simulink model "cichbcic_core"  (Simulink 7.9)
settings: Solver=ode45  StartTime=0.0  StopTime=10.0  RelTol=1e-3
libraries: xbsIndex_r4 x375
(part 2 of 5)

== system cichbcic_core/cic_stage_dec4/adder_tree1 ==
  sync : Inport
  din_1 : Inport  Port=2
  din_2 : Inport  Port=3
  adder_0 : xbsIndex_r4/AddSub  mode=Addition  use_carryin=off  use_carryout=off  en=off  latency=4  precision=Full  arith_type=Unsigned  n_bits=18  bin_pt=17  quantization="Round  (unbiased: +/- Inf)"  overflow=Saturate  dbl_ovrd=off  use_behavioral_HDL=on  hw_selection=Fabric  pipelined=off  block_type=addsub
  sync_delay : xbsIndex_r4/Delay  rst=off  infoeditControl=Selection of Reset will increase slice count due to use of real FFs and instead of SRLs  en=off  latency=4  dbl_ovrd=off  reg_retiming=off  block_type=delay
  sync_out : Outport
  dout : Outport  Port=2
  wires:
  sync/1 -> sync_delay/1
  sync_delay/1 -> sync_out/1
  din_2/1 -> adder_0/1
  din_1/1 -> adder_0/2
  adder_0/1 -> dout/1

== system cichbcic_core/cic_stage_dec4/adder_tree2 ==
  sync : Inport
  din_1 : Inport  Port=2
  din_2 : Inport  Port=3
  adder_0 : xbsIndex_r4/AddSub  mode=Addition  use_carryin=off  use_carryout=off  en=off  latency=4  precision=Full  arith_type=Unsigned  n_bits=18  bin_pt=17  quantization="Round  (unbiased: +/- Inf)"  overflow=Saturate  dbl_ovrd=off  use_behavioral_HDL=on  hw_selection=Fabric  pipelined=off  block_type=addsub
  sync_delay : xbsIndex_r4/Delay  rst=off  infoeditControl=Selection of Reset will increase slice count due to use of real FFs and instead of SRLs  en=off  latency=4  dbl_ovrd=off  reg_retiming=off  block_type=delay
  sync_out : Outport
  dout : Outport  Port=2
  wires:
  sync/1 -> sync_delay/1
  sync_delay/1 -> sync_out/1
  din_2/1 -> adder_0/1
  din_1/1 -> adder_0/2
  adder_0/1 -> dout/1

== system cichbcic_core/cic_stage_dec4/adder_tree3 ==
  sync : Inport
  din_1 : Inport  Port=2
  din_2 : Inport  Port=3
  adder_0 : xbsIndex_r4/AddSub  mode=Addition  use_carryin=off  use_carryout=off  en=off  latency=4  precision=Full  arith_type=Unsigned  n_bits=18  bin_pt=17  quantization="Round  (unbiased: +/- Inf)"  overflow=Saturate  dbl_ovrd=off  use_behavioral_HDL=on  hw_selection=Fabric  pipelined=off  block_type=addsub
  sync_delay : xbsIndex_r4/Delay  rst=off  infoeditControl=Selection of Reset will increase slice count due to use of real FFs and instead of SRLs  en=off  latency=4  dbl_ovrd=off  reg_retiming=off  block_type=delay
  sync_out : Outport
  dout : Outport  Port=2
  wires:
  sync/1 -> sync_delay/1
  sync_delay/1 -> sync_out/1
  din_2/1 -> adder_0/1
  din_1/1 -> adder_0/2
  adder_0/1 -> dout/1

== system cichbcic_core/Halfband1/adder_tree/addr1 ==
  data_a : Inport
  data_b : Inport  Port=2
  en_in : Inport  Port=3
  AddSub : xbsIndex_r4/AddSub  mode=Addition  use_carryin=off  use_carryout=off  en=on  latency=2  precision=Full  arith_type=Unsigned  n_bits=16  bin_pt=14  quantization=Truncate  overflow=Wrap  dbl_ovrd=off  use_behavioral_HDL=off  hw_selection=Fabric  pipelined=off  block_type=addsub
  sum_ab : Outport
  en_out : Outport  Port=2
  wires:
  data_b/1 -> AddSub/1
  data_a/1 -> AddSub/2
  en_in/1 -> AddSub/3, en_out/1
  AddSub/1 -> sum_ab/1

== system cichbcic_core/Halfband1/adder_tree/addr11 ==
  data_a : Inport
  data_b : Inport  Port=2
  en_in : Inport  Port=3
  AddSub : xbsIndex_r4/AddSub  mode=Addition  use_carryin=off  use_carryout=off  en=on  latency=2  precision=Full  arith_type=Unsigned  n_bits=16  bin_pt=14  quantization=Truncate  overflow=Wrap  dbl_ovrd=off  use_behavioral_HDL=off  hw_selection=Fabric  pipelined=off  block_type=addsub
  sum_ab : Outport
  en_out : Outport  Port=2
  wires:
  data_b/1 -> AddSub/1
  data_a/1 -> AddSub/2
  en_in/1 -> AddSub/3, en_out/1
  AddSub/1 -> sum_ab/1

== system cichbcic_core/Halfband1/adder_tree/addr2 ==
  data_a : Inport
  data_b : Inport  Port=2
  en_in : Inport  Port=3
  AddSub : xbsIndex_r4/AddSub  mode=Addition  use_carryin=off  use_carryout=off  en=on  latency=2  precision=Full  arith_type=Unsigned  n_bits=16  bin_pt=14  quantization=Truncate  overflow=Wrap  dbl_ovrd=off  use_behavioral_HDL=off  hw_selection=Fabric  pipelined=off  block_type=addsub
  sum_ab : Outport
  en_out : Outport  Port=2
  wires:
  data_b/1 -> AddSub/1
  data_a/1 -> AddSub/2
  en_in/1 -> AddSub/3, en_out/1
  AddSub/1 -> sum_ab/1

== system cichbcic_core/Halfband1/adder_tree/addr3 ==
  data_a : Inport
  data_b : Inport  Port=2
  en_in : Inport  Port=3
  AddSub : xbsIndex_r4/AddSub  mode=Addition  use_carryin=off  use_carryout=off  en=on  latency=2  precision=Full  arith_type=Unsigned  n_bits=16  bin_pt=14  quantization=Truncate  overflow=Wrap  dbl_ovrd=off  use_behavioral_HDL=off  hw_selection=Fabric  pipelined=off  block_type=addsub
  sum_ab : Outport
  en_out : Outport  Port=2
  wires:
  data_b/1 -> AddSub/1
  data_a/1 -> AddSub/2
  en_in/1 -> AddSub/3, en_out/1
  AddSub/1 -> sum_ab/1

== system cichbcic_core/Halfband1/adder_tree/addr4 ==
  data_a : Inport
  data_b : Inport  Port=2
  en_in : Inport  Port=3
  AddSub : xbsIndex_r4/AddSub  mode=Addition  use_carryin=off  use_carryout=off  en=on  latency=2  precision=Full  arith_type=Unsigned  n_bits=16  bin_pt=14  quantization=Truncate  overflow=Wrap  dbl_ovrd=off  use_behavioral_HDL=off  hw_selection=Fabric  pipelined=off  block_type=addsub
  sum_ab : Outport
  en_out : Outport  Port=2
  wires:
  data_b/1 -> AddSub/1
  data_a/1 -> AddSub/2
  en_in/1 -> AddSub/3, en_out/1
  AddSub/1 -> sum_ab/1

== system cichbcic_core/Halfband1/adder_tree/addr6 ==
  data_a : Inport
  data_b : Inport  Port=2
  en_in : Inport  Port=3
  AddSub : xbsIndex_r4/AddSub  mode=Addition  use_carryin=off  use_carryout=off  en=on  latency=2  precision=Full  arith_type=Unsigned  n_bits=16  bin_pt=14  quantization=Truncate  overflow=Wrap  dbl_ovrd=off  use_behavioral_HDL=off  hw_selection=Fabric  pipelined=off  block_type=addsub
  sum_ab : Outport
  en_out : Outport  Port=2
  wires:
  data_b/1 -> AddSub/1
  data_a/1 -> AddSub/2
  en_in/1 -> AddSub/3, en_out/1
  AddSub/1 -> sum_ab/1

== system cichbcic_core/Halfband1/adder_tree/addr7 ==
  data_a : Inport
  data_b : Inport  Port=2
  en_in : Inport  Port=3
  AddSub : xbsIndex_r4/AddSub  mode=Addition  use_carryin=off  use_carryout=off  en=on  latency=2  precision=Full  arith_type=Unsigned  n_bits=16  bin_pt=14  quantization=Truncate  overflow=Wrap  dbl_ovrd=off  use_behavioral_HDL=off  hw_selection=Fabric  pipelined=off  block_type=addsub
  sum_ab : Outport
  en_out : Outport  Port=2
  wires:
  data_b/1 -> AddSub/1
  data_a/1 -> AddSub/2
  en_in/1 -> AddSub/3, en_out/1
  AddSub/1 -> sum_ab/1

== system cichbcic_core/Halfband1/adder_tree/addr9 ==
  data_a : Inport
  data_b : Inport  Port=2
  en_in : Inport  Port=3
  AddSub : xbsIndex_r4/AddSub  mode=Addition  use_carryin=off  use_carryout=off  en=on  latency=2  precision=Full  arith_type=Unsigned  n_bits=16  bin_pt=14  quantization=Truncate  overflow=Wrap  dbl_ovrd=off  use_behavioral_HDL=off  hw_selection=Fabric  pipelined=off  block_type=addsub
  sum_ab : Outport
  en_out : Outport  Port=2
  wires:
  data_b/1 -> AddSub/1
  data_a/1 -> AddSub/2
  en_in/1 -> AddSub/3, en_out/1
  AddSub/1 -> sum_ab/1

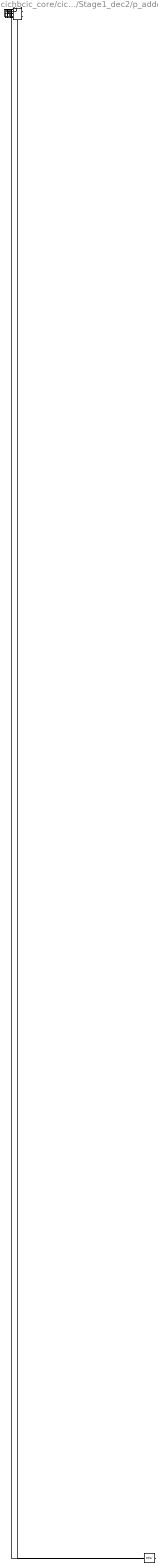
== system cichbcic_core/cic_pow2_1/Stage1_dec2/p_adder1 ==
  sync_in : Inport
  in1 : Inport  Port=2
  in2 : Inport  Port=3
  in3 : Inport  Port=4
  in4 : Inport  Port=5
  in5 : Inport  Port=6
  in6 : Inport  Port=7
  in7 : Inport  Port=8
  in8 : Inport  Port=9
  in9 : Inport  Port=10
  in10 : Inport  Port=11
  in11 : Inport  Port=12
  in12 : Inport  Port=13
  in13 : Inport  Port=14
  in14 : Inport  Port=15
  in15 : Inport  Port=16
  in16 : Inport  Port=17
  adder_tree1 : Subsystem
  adder_tree10 : Subsystem
  adder_tree11 : Subsystem
  adder_tree12 : Subsystem
  adder_tree13 : Subsystem
  adder_tree14 : Subsystem
  adder_tree15 : Subsystem
  adder_tree16 : Subsystem
  adder_tree2 : Subsystem
  adder_tree3 : Subsystem
  adder_tree4 : Subsystem
  adder_tree5 : Subsystem
  adder_tree6 : Subsystem
  adder_tree7 : Subsystem
  adder_tree8 : Subsystem
  adder_tree9 : Subsystem
  delay16 : xbsIndex_r4/Delay  rst=off  infoeditControl=Selection of Reset will increase slice count due to use of real FFs and instead of SRLs  en=off  latency=1  dbl_ovrd=off  reg_retiming=off  block_type=delay
  sync_out : Outport
  out1 : Outport  Port=2
  out2 : Outport  Port=3
  out3 : Outport  Port=4
  out4 : Outport  Port=5
  out5 : Outport  Port=6
  out6 : Outport  Port=7
  out7 : Outport  Port=8
  out8 : Outport  Port=9
  out9 : Outport  Port=10
  out10 : Outport  Port=11
  out11 : Outport  Port=12
  out12 : Outport  Port=13
  out13 : Outport  Port=14
  out14 : Outport  Port=15
  out15 : Outport  Port=16
  out16 : Outport  Port=17
  wires:
  in16/1 -> delay16/1, adder_tree16/2(din_1)
  sync_in/1 -> adder_tree1/1(sync)
  in1/1 -> adder_tree1/2(din_1), adder_tree2/3(din_2)
  delay16/1 -> adder_tree1/3(din_2)  "d16"
  adder_tree1/2(dout) -> out1/1
  adder_tree1/1(sync_out) -> adder_tree2/1(sync)  "adder_tree_sync_in1"
  in2/1 -> adder_tree2/2(din_1), adder_tree3/3(din_2)
  adder_tree2/2(dout) -> out2/1
  adder_tree2/1(sync_out) -> adder_tree3/1(sync)  "adder_tree_sync_in2"
  in3/1 -> adder_tree3/2(din_1), adder_tree4/3(din_2)
  adder_tree3/2(dout) -> out3/1
  adder_tree3/1(sync_out) -> adder_tree4/1(sync)  "adder_tree_sync_in3"
  in4/1 -> adder_tree4/2(din_1), adder_tree5/3(din_2)
  adder_tree4/2(dout) -> out4/1
  adder_tree4/1(sync_out) -> adder_tree5/1(sync)  "adder_tree_sync_in4"
  in5/1 -> adder_tree5/2(din_1), adder_tree6/3(din_2)
  adder_tree5/2(dout) -> out5/1
  adder_tree5/1(sync_out) -> adder_tree6/1(sync)  "adder_tree_sync_in5"
  in6/1 -> adder_tree6/2(din_1), adder_tree7/3(din_2)
  adder_tree6/2(dout) -> out6/1
  adder_tree6/1(sync_out) -> adder_tree7/1(sync)  "adder_tree_sync_in6"
  in7/1 -> adder_tree7/2(din_1), adder_tree8/3(din_2)
  adder_tree7/2(dout) -> out7/1
  adder_tree7/1(sync_out) -> adder_tree8/1(sync)  "adder_tree_sync_in7"
  in8/1 -> adder_tree8/2(din_1), adder_tree9/3(din_2)
  adder_tree8/2(dout) -> out8/1
  adder_tree8/1(sync_out) -> adder_tree9/1(sync)  "adder_tree_sync_in8"
  in9/1 -> adder_tree9/2(din_1), adder_tree10/3(din_2)
  adder_tree9/2(dout) -> out9/1
  adder_tree9/1(sync_out) -> adder_tree10/1(sync)  "adder_tree_sync_in9"
  in10/1 -> adder_tree10/2(din_1), adder_tree11/3(din_2)
  adder_tree10/2(dout) -> out10/1
  adder_tree10/1(sync_out) -> adder_tree11/1(sync)  "adder_tree_sync_in10"
  in11/1 -> adder_tree11/2(din_1), adder_tree12/3(din_2)
  adder_tree11/2(dout) -> out11/1
  adder_tree11/1(sync_out) -> adder_tree12/1(sync)  "adder_tree_sync_in11"
  in12/1 -> adder_tree12/2(din_1), adder_tree13/3(din_2)
  adder_tree12/2(dout) -> out12/1
  adder_tree12/1(sync_out) -> adder_tree13/1(sync)  "adder_tree_sync_in12"
  in13/1 -> adder_tree13/2(din_1), adder_tree14/3(din_2)
  adder_tree13/2(dout) -> out13/1
  adder_tree13/1(sync_out) -> adder_tree14/1(sync)  "adder_tree_sync_in13"
  in14/1 -> adder_tree14/2(din_1), adder_tree15/3(din_2)
  adder_tree14/2(dout) -> out14/1
  adder_tree14/1(sync_out) -> adder_tree15/1(sync)  "adder_tree_sync_in14"
  in15/1 -> adder_tree15/2(din_1), adder_tree16/3(din_2)
  adder_tree15/2(dout) -> out15/1
  adder_tree15/1(sync_out) -> adder_tree16/1(sync)  "adder_tree_sync_in15"
  adder_tree16/2(dout) -> out16/1
  adder_tree16/1(sync_out) -> sync_out/1  "adder_tree_sync_in16"

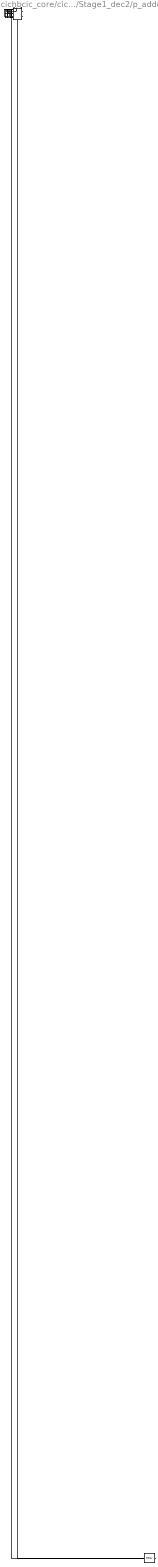
== system cichbcic_core/cic_pow2_1/Stage1_dec2/p_adder2 ==
  sync_in : Inport
  in1 : Inport  Port=2
  in2 : Inport  Port=3
  in3 : Inport  Port=4
  in4 : Inport  Port=5
  in5 : Inport  Port=6
  in6 : Inport  Port=7
  in7 : Inport  Port=8
  in8 : Inport  Port=9
  in9 : Inport  Port=10
  in10 : Inport  Port=11
  in11 : Inport  Port=12
  in12 : Inport  Port=13
  in13 : Inport  Port=14
  in14 : Inport  Port=15
  in15 : Inport  Port=16
  in16 : Inport  Port=17
  adder_tree1 : Subsystem
  adder_tree10 : Subsystem
  adder_tree11 : Subsystem
  adder_tree12 : Subsystem
  adder_tree13 : Subsystem
  adder_tree14 : Subsystem
  adder_tree15 : Subsystem
  adder_tree16 : Subsystem
  adder_tree2 : Subsystem
  adder_tree3 : Subsystem
  adder_tree4 : Subsystem
  adder_tree5 : Subsystem
  adder_tree6 : Subsystem
  adder_tree7 : Subsystem
  adder_tree8 : Subsystem
  adder_tree9 : Subsystem
  delay16 : xbsIndex_r4/Delay  rst=off  infoeditControl=Selection of Reset will increase slice count due to use of real FFs and instead of SRLs  en=off  latency=1  dbl_ovrd=off  reg_retiming=off  block_type=delay
  sync_out : Outport
  out1 : Outport  Port=2
  out2 : Outport  Port=3
  out3 : Outport  Port=4
  out4 : Outport  Port=5
  out5 : Outport  Port=6
  out6 : Outport  Port=7
  out7 : Outport  Port=8
  out8 : Outport  Port=9
  out9 : Outport  Port=10
  out10 : Outport  Port=11
  out11 : Outport  Port=12
  out12 : Outport  Port=13
  out13 : Outport  Port=14
  out14 : Outport  Port=15
  out15 : Outport  Port=16
  out16 : Outport  Port=17
  wires:
  in16/1 -> delay16/1, adder_tree16/2(din_1)
  sync_in/1 -> adder_tree1/1(sync)
  in1/1 -> adder_tree1/2(din_1), adder_tree2/3(din_2)
  delay16/1 -> adder_tree1/3(din_2)  "d16"
  adder_tree1/2(dout) -> out1/1
  adder_tree1/1(sync_out) -> adder_tree2/1(sync)  "adder_tree_sync_in1"
  in2/1 -> adder_tree2/2(din_1), adder_tree3/3(din_2)
  adder_tree2/2(dout) -> out2/1
  adder_tree2/1(sync_out) -> adder_tree3/1(sync)  "adder_tree_sync_in2"
  in3/1 -> adder_tree3/2(din_1), adder_tree4/3(din_2)
  adder_tree3/2(dout) -> out3/1
  adder_tree3/1(sync_out) -> adder_tree4/1(sync)  "adder_tree_sync_in3"
  in4/1 -> adder_tree4/2(din_1), adder_tree5/3(din_2)
  adder_tree4/2(dout) -> out4/1
  adder_tree4/1(sync_out) -> adder_tree5/1(sync)  "adder_tree_sync_in4"
  in5/1 -> adder_tree5/2(din_1), adder_tree6/3(din_2)
  adder_tree5/2(dout) -> out5/1
  adder_tree5/1(sync_out) -> adder_tree6/1(sync)  "adder_tree_sync_in5"
  in6/1 -> adder_tree6/2(din_1), adder_tree7/3(din_2)
  adder_tree6/2(dout) -> out6/1
  adder_tree6/1(sync_out) -> adder_tree7/1(sync)  "adder_tree_sync_in6"
  in7/1 -> adder_tree7/2(din_1), adder_tree8/3(din_2)
  adder_tree7/2(dout) -> out7/1
  adder_tree7/1(sync_out) -> adder_tree8/1(sync)  "adder_tree_sync_in7"
  in8/1 -> adder_tree8/2(din_1), adder_tree9/3(din_2)
  adder_tree8/2(dout) -> out8/1
  adder_tree8/1(sync_out) -> adder_tree9/1(sync)  "adder_tree_sync_in8"
  in9/1 -> adder_tree9/2(din_1), adder_tree10/3(din_2)
  adder_tree9/2(dout) -> out9/1
  adder_tree9/1(sync_out) -> adder_tree10/1(sync)  "adder_tree_sync_in9"
  in10/1 -> adder_tree10/2(din_1), adder_tree11/3(din_2)
  adder_tree10/2(dout) -> out10/1
  adder_tree10/1(sync_out) -> adder_tree11/1(sync)  "adder_tree_sync_in10"
  in11/1 -> adder_tree11/2(din_1), adder_tree12/3(din_2)
  adder_tree11/2(dout) -> out11/1
  adder_tree11/1(sync_out) -> adder_tree12/1(sync)  "adder_tree_sync_in11"
  in12/1 -> adder_tree12/2(din_1), adder_tree13/3(din_2)
  adder_tree12/2(dout) -> out12/1
  adder_tree12/1(sync_out) -> adder_tree13/1(sync)  "adder_tree_sync_in12"
  in13/1 -> adder_tree13/2(din_1), adder_tree14/3(din_2)
  adder_tree13/2(dout) -> out13/1
  adder_tree13/1(sync_out) -> adder_tree14/1(sync)  "adder_tree_sync_in13"
  in14/1 -> adder_tree14/2(din_1), adder_tree15/3(din_2)
  adder_tree14/2(dout) -> out14/1
  adder_tree14/1(sync_out) -> adder_tree15/1(sync)  "adder_tree_sync_in14"
  in15/1 -> adder_tree15/2(din_1), adder_tree16/3(din_2)
  adder_tree15/2(dout) -> out15/1
  adder_tree15/1(sync_out) -> adder_tree16/1(sync)  "adder_tree_sync_in15"
  adder_tree16/2(dout) -> out16/1
  adder_tree16/1(sync_out) -> sync_out/1  "adder_tree_sync_in16"

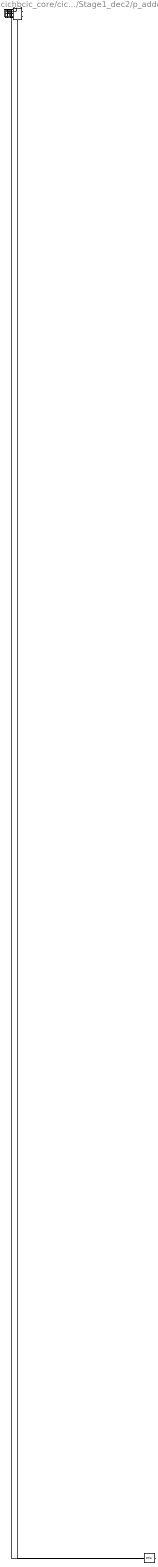
== system cichbcic_core/cic_pow2_1/Stage1_dec2/p_adder3 ==
  sync_in : Inport
  in1 : Inport  Port=2
  in2 : Inport  Port=3
  in3 : Inport  Port=4
  in4 : Inport  Port=5
  in5 : Inport  Port=6
  in6 : Inport  Port=7
  in7 : Inport  Port=8
  in8 : Inport  Port=9
  in9 : Inport  Port=10
  in10 : Inport  Port=11
  in11 : Inport  Port=12
  in12 : Inport  Port=13
  in13 : Inport  Port=14
  in14 : Inport  Port=15
  in15 : Inport  Port=16
  in16 : Inport  Port=17
  adder_tree1 : Subsystem
  adder_tree10 : Subsystem
  adder_tree11 : Subsystem
  adder_tree12 : Subsystem
  adder_tree13 : Subsystem
  adder_tree14 : Subsystem
  adder_tree15 : Subsystem
  adder_tree16 : Subsystem
  adder_tree2 : Subsystem
  adder_tree3 : Subsystem
  adder_tree4 : Subsystem
  adder_tree5 : Subsystem
  adder_tree6 : Subsystem
  adder_tree7 : Subsystem
  adder_tree8 : Subsystem
  adder_tree9 : Subsystem
  delay16 : xbsIndex_r4/Delay  rst=off  infoeditControl=Selection of Reset will increase slice count due to use of real FFs and instead of SRLs  en=off  latency=1  dbl_ovrd=off  reg_retiming=off  block_type=delay
  sync_out : Outport
  out1 : Outport  Port=2
  out2 : Outport  Port=3
  out3 : Outport  Port=4
  out4 : Outport  Port=5
  out5 : Outport  Port=6
  out6 : Outport  Port=7
  out7 : Outport  Port=8
  out8 : Outport  Port=9
  out9 : Outport  Port=10
  out10 : Outport  Port=11
  out11 : Outport  Port=12
  out12 : Outport  Port=13
  out13 : Outport  Port=14
  out14 : Outport  Port=15
  out15 : Outport  Port=16
  out16 : Outport  Port=17
  wires:
  in16/1 -> delay16/1, adder_tree16/2(din_1)
  sync_in/1 -> adder_tree1/1(sync)
  in1/1 -> adder_tree1/2(din_1), adder_tree2/3(din_2)
  delay16/1 -> adder_tree1/3(din_2)  "d16"
  adder_tree1/2(dout) -> out1/1
  adder_tree1/1(sync_out) -> adder_tree2/1(sync)  "adder_tree_sync_in1"
  in2/1 -> adder_tree2/2(din_1), adder_tree3/3(din_2)
  adder_tree2/2(dout) -> out2/1
  adder_tree2/1(sync_out) -> adder_tree3/1(sync)  "adder_tree_sync_in2"
  in3/1 -> adder_tree3/2(din_1), adder_tree4/3(din_2)
  adder_tree3/2(dout) -> out3/1
  adder_tree3/1(sync_out) -> adder_tree4/1(sync)  "adder_tree_sync_in3"
  in4/1 -> adder_tree4/2(din_1), adder_tree5/3(din_2)
  adder_tree4/2(dout) -> out4/1
  adder_tree4/1(sync_out) -> adder_tree5/1(sync)  "adder_tree_sync_in4"
  in5/1 -> adder_tree5/2(din_1), adder_tree6/3(din_2)
  adder_tree5/2(dout) -> out5/1
  adder_tree5/1(sync_out) -> adder_tree6/1(sync)  "adder_tree_sync_in5"
  in6/1 -> adder_tree6/2(din_1), adder_tree7/3(din_2)
  adder_tree6/2(dout) -> out6/1
  adder_tree6/1(sync_out) -> adder_tree7/1(sync)  "adder_tree_sync_in6"
  in7/1 -> adder_tree7/2(din_1), adder_tree8/3(din_2)
  adder_tree7/2(dout) -> out7/1
  adder_tree7/1(sync_out) -> adder_tree8/1(sync)  "adder_tree_sync_in7"
  in8/1 -> adder_tree8/2(din_1), adder_tree9/3(din_2)
  adder_tree8/2(dout) -> out8/1
  adder_tree8/1(sync_out) -> adder_tree9/1(sync)  "adder_tree_sync_in8"
  in9/1 -> adder_tree9/2(din_1), adder_tree10/3(din_2)
  adder_tree9/2(dout) -> out9/1
  adder_tree9/1(sync_out) -> adder_tree10/1(sync)  "adder_tree_sync_in9"
  in10/1 -> adder_tree10/2(din_1), adder_tree11/3(din_2)
  adder_tree10/2(dout) -> out10/1
  adder_tree10/1(sync_out) -> adder_tree11/1(sync)  "adder_tree_sync_in10"
  in11/1 -> adder_tree11/2(din_1), adder_tree12/3(din_2)
  adder_tree11/2(dout) -> out11/1
  adder_tree11/1(sync_out) -> adder_tree12/1(sync)  "adder_tree_sync_in11"
  in12/1 -> adder_tree12/2(din_1), adder_tree13/3(din_2)
  adder_tree12/2(dout) -> out12/1
  adder_tree12/1(sync_out) -> adder_tree13/1(sync)  "adder_tree_sync_in12"
  in13/1 -> adder_tree13/2(din_1), adder_tree14/3(din_2)
  adder_tree13/2(dout) -> out13/1
  adder_tree13/1(sync_out) -> adder_tree14/1(sync)  "adder_tree_sync_in13"
  in14/1 -> adder_tree14/2(din_1), adder_tree15/3(din_2)
  adder_tree14/2(dout) -> out14/1
  adder_tree14/1(sync_out) -> adder_tree15/1(sync)  "adder_tree_sync_in14"
  in15/1 -> adder_tree15/2(din_1), adder_tree16/3(din_2)
  adder_tree15/2(dout) -> out15/1
  adder_tree15/1(sync_out) -> adder_tree16/1(sync)  "adder_tree_sync_in15"
  adder_tree16/2(dout) -> out16/1
  adder_tree16/1(sync_out) -> sync_out/1  "adder_tree_sync_in16"

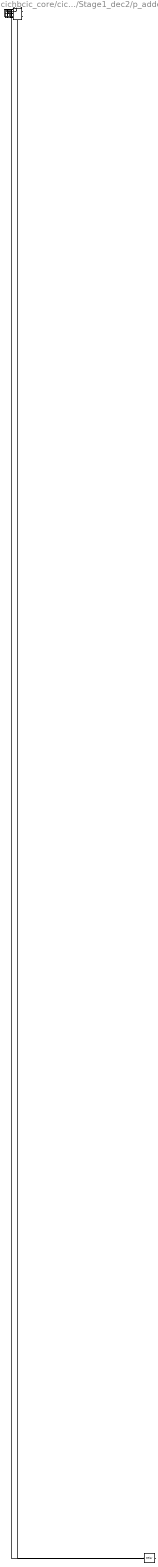
== system cichbcic_core/cic_pow2_1/Stage1_dec2/p_adder4 ==
  sync_in : Inport
  in1 : Inport  Port=2
  in2 : Inport  Port=3
  in3 : Inport  Port=4
  in4 : Inport  Port=5
  in5 : Inport  Port=6
  in6 : Inport  Port=7
  in7 : Inport  Port=8
  in8 : Inport  Port=9
  in9 : Inport  Port=10
  in10 : Inport  Port=11
  in11 : Inport  Port=12
  in12 : Inport  Port=13
  in13 : Inport  Port=14
  in14 : Inport  Port=15
  in15 : Inport  Port=16
  in16 : Inport  Port=17
  adder_tree1 : Subsystem
  adder_tree10 : Subsystem
  adder_tree11 : Subsystem
  adder_tree12 : Subsystem
  adder_tree13 : Subsystem
  adder_tree14 : Subsystem
  adder_tree15 : Subsystem
  adder_tree16 : Subsystem
  adder_tree2 : Subsystem
  adder_tree3 : Subsystem
  adder_tree4 : Subsystem
  adder_tree5 : Subsystem
  adder_tree6 : Subsystem
  adder_tree7 : Subsystem
  adder_tree8 : Subsystem
  adder_tree9 : Subsystem
  delay16 : xbsIndex_r4/Delay  rst=off  infoeditControl=Selection of Reset will increase slice count due to use of real FFs and instead of SRLs  en=off  latency=1  dbl_ovrd=off  reg_retiming=off  block_type=delay
  sync_out : Outport
  out1 : Outport  Port=2
  out2 : Outport  Port=3
  out3 : Outport  Port=4
  out4 : Outport  Port=5
  out5 : Outport  Port=6
  out6 : Outport  Port=7
  out7 : Outport  Port=8
  out8 : Outport  Port=9
  out9 : Outport  Port=10
  out10 : Outport  Port=11
  out11 : Outport  Port=12
  out12 : Outport  Port=13
  out13 : Outport  Port=14
  out14 : Outport  Port=15
  out15 : Outport  Port=16
  out16 : Outport  Port=17
  wires:
  in16/1 -> delay16/1, adder_tree16/2(din_1)
  sync_in/1 -> adder_tree1/1(sync)
  in1/1 -> adder_tree1/2(din_1), adder_tree2/3(din_2)
  delay16/1 -> adder_tree1/3(din_2)  "d16"
  adder_tree1/2(dout) -> out1/1
  adder_tree1/1(sync_out) -> adder_tree2/1(sync)  "adder_tree_sync_in1"
  in2/1 -> adder_tree2/2(din_1), adder_tree3/3(din_2)
  adder_tree2/2(dout) -> out2/1
  adder_tree2/1(sync_out) -> adder_tree3/1(sync)  "adder_tree_sync_in2"
  in3/1 -> adder_tree3/2(din_1), adder_tree4/3(din_2)
  adder_tree3/2(dout) -> out3/1
  adder_tree3/1(sync_out) -> adder_tree4/1(sync)  "adder_tree_sync_in3"
  in4/1 -> adder_tree4/2(din_1), adder_tree5/3(din_2)
  adder_tree4/2(dout) -> out4/1
  adder_tree4/1(sync_out) -> adder_tree5/1(sync)  "adder_tree_sync_in4"
  in5/1 -> adder_tree5/2(din_1), adder_tree6/3(din_2)
  adder_tree5/2(dout) -> out5/1
  adder_tree5/1(sync_out) -> adder_tree6/1(sync)  "adder_tree_sync_in5"
  in6/1 -> adder_tree6/2(din_1), adder_tree7/3(din_2)
  adder_tree6/2(dout) -> out6/1
  adder_tree6/1(sync_out) -> adder_tree7/1(sync)  "adder_tree_sync_in6"
  in7/1 -> adder_tree7/2(din_1), adder_tree8/3(din_2)
  adder_tree7/2(dout) -> out7/1
  adder_tree7/1(sync_out) -> adder_tree8/1(sync)  "adder_tree_sync_in7"
  in8/1 -> adder_tree8/2(din_1), adder_tree9/3(din_2)
  adder_tree8/2(dout) -> out8/1
  adder_tree8/1(sync_out) -> adder_tree9/1(sync)  "adder_tree_sync_in8"
  in9/1 -> adder_tree9/2(din_1), adder_tree10/3(din_2)
  adder_tree9/2(dout) -> out9/1
  adder_tree9/1(sync_out) -> adder_tree10/1(sync)  "adder_tree_sync_in9"
  in10/1 -> adder_tree10/2(din_1), adder_tree11/3(din_2)
  adder_tree10/2(dout) -> out10/1
  adder_tree10/1(sync_out) -> adder_tree11/1(sync)  "adder_tree_sync_in10"
  in11/1 -> adder_tree11/2(din_1), adder_tree12/3(din_2)
  adder_tree11/2(dout) -> out11/1
  adder_tree11/1(sync_out) -> adder_tree12/1(sync)  "adder_tree_sync_in11"
  in12/1 -> adder_tree12/2(din_1), adder_tree13/3(din_2)
  adder_tree12/2(dout) -> out12/1
  adder_tree12/1(sync_out) -> adder_tree13/1(sync)  "adder_tree_sync_in12"
  in13/1 -> adder_tree13/2(din_1), adder_tree14/3(din_2)
  adder_tree13/2(dout) -> out13/1
  adder_tree13/1(sync_out) -> adder_tree14/1(sync)  "adder_tree_sync_in13"
  in14/1 -> adder_tree14/2(din_1), adder_tree15/3(din_2)
  adder_tree14/2(dout) -> out14/1
  adder_tree14/1(sync_out) -> adder_tree15/1(sync)  "adder_tree_sync_in14"
  in15/1 -> adder_tree15/2(din_1), adder_tree16/3(din_2)
  adder_tree15/2(dout) -> out15/1
  adder_tree15/1(sync_out) -> adder_tree16/1(sync)  "adder_tree_sync_in15"
  adder_tree16/2(dout) -> out16/1
  adder_tree16/1(sync_out) -> sync_out/1  "adder_tree_sync_in16"

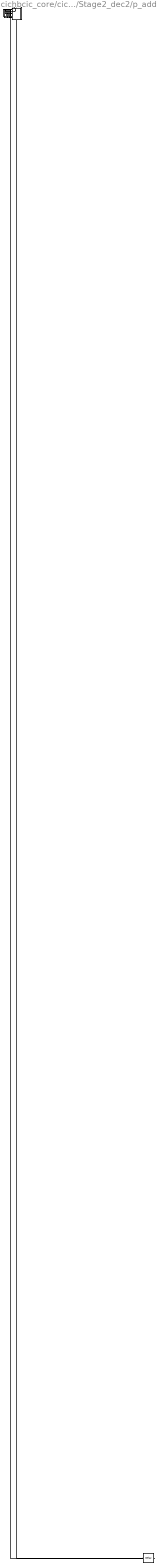
== system cichbcic_core/cic_pow2_1/Stage2_dec2/p_adder1 ==
  sync_in : Inport
  in1 : Inport  Port=2
  in2 : Inport  Port=3
  in3 : Inport  Port=4
  in4 : Inport  Port=5
  in5 : Inport  Port=6
  in6 : Inport  Port=7
  in7 : Inport  Port=8
  in8 : Inport  Port=9
  adder_tree1 : Subsystem
  adder_tree2 : Subsystem
  adder_tree3 : Subsystem
  adder_tree4 : Subsystem
  adder_tree5 : Subsystem
  adder_tree6 : Subsystem
  adder_tree7 : Subsystem
  adder_tree8 : Subsystem
  delay8 : xbsIndex_r4/Delay  rst=off  infoeditControl=Selection of Reset will increase slice count due to use of real FFs and instead of SRLs  en=off  latency=1  dbl_ovrd=off  reg_retiming=off  block_type=delay
  sync_out : Outport
  out1 : Outport  Port=2
  out2 : Outport  Port=3
  out3 : Outport  Port=4
  out4 : Outport  Port=5
  out5 : Outport  Port=6
  out6 : Outport  Port=7
  out7 : Outport  Port=8
  out8 : Outport  Port=9
  wires:
  in8/1 -> delay8/1, adder_tree8/2(din_1)
  sync_in/1 -> adder_tree1/1(sync)
  in1/1 -> adder_tree1/2(din_1), adder_tree2/3(din_2)
  delay8/1 -> adder_tree1/3(din_2)  "d8"
  adder_tree1/2(dout) -> out1/1
  adder_tree1/1(sync_out) -> adder_tree2/1(sync)  "adder_tree_sync_in1"
  in2/1 -> adder_tree2/2(din_1), adder_tree3/3(din_2)
  adder_tree2/2(dout) -> out2/1
  adder_tree2/1(sync_out) -> adder_tree3/1(sync)  "adder_tree_sync_in2"
  in3/1 -> adder_tree3/2(din_1), adder_tree4/3(din_2)
  adder_tree3/2(dout) -> out3/1
  adder_tree3/1(sync_out) -> adder_tree4/1(sync)  "adder_tree_sync_in3"
  in4/1 -> adder_tree4/2(din_1), adder_tree5/3(din_2)
  adder_tree4/2(dout) -> out4/1
  adder_tree4/1(sync_out) -> adder_tree5/1(sync)  "adder_tree_sync_in4"
  in5/1 -> adder_tree5/2(din_1), adder_tree6/3(din_2)
  adder_tree5/2(dout) -> out5/1
  adder_tree5/1(sync_out) -> adder_tree6/1(sync)  "adder_tree_sync_in5"
  in6/1 -> adder_tree6/2(din_1), adder_tree7/3(din_2)
  adder_tree6/2(dout) -> out6/1
  adder_tree6/1(sync_out) -> adder_tree7/1(sync)  "adder_tree_sync_in6"
  in7/1 -> adder_tree7/2(din_1), adder_tree8/3(din_2)
  adder_tree7/2(dout) -> out7/1
  adder_tree7/1(sync_out) -> adder_tree8/1(sync)  "adder_tree_sync_in7"
  adder_tree8/2(dout) -> out8/1
  adder_tree8/1(sync_out) -> sync_out/1  "adder_tree_sync_in8"

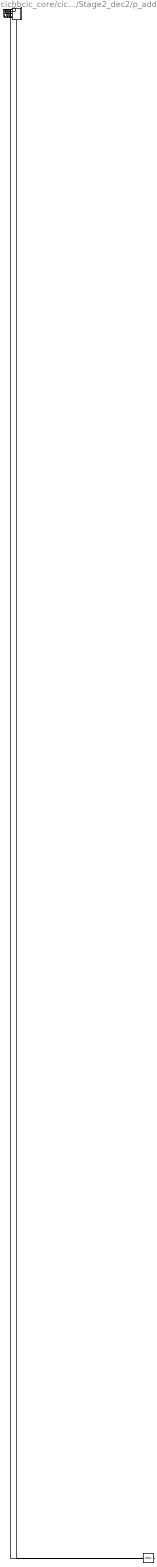
== system cichbcic_core/cic_pow2_1/Stage2_dec2/p_adder2 ==
  sync_in : Inport
  in1 : Inport  Port=2
  in2 : Inport  Port=3
  in3 : Inport  Port=4
  in4 : Inport  Port=5
  in5 : Inport  Port=6
  in6 : Inport  Port=7
  in7 : Inport  Port=8
  in8 : Inport  Port=9
  adder_tree1 : Subsystem
  adder_tree2 : Subsystem
  adder_tree3 : Subsystem
  adder_tree4 : Subsystem
  adder_tree5 : Subsystem
  adder_tree6 : Subsystem
  adder_tree7 : Subsystem
  adder_tree8 : Subsystem
  delay8 : xbsIndex_r4/Delay  rst=off  infoeditControl=Selection of Reset will increase slice count due to use of real FFs and instead of SRLs  en=off  latency=1  dbl_ovrd=off  reg_retiming=off  block_type=delay
  sync_out : Outport
  out1 : Outport  Port=2
  out2 : Outport  Port=3
  out3 : Outport  Port=4
  out4 : Outport  Port=5
  out5 : Outport  Port=6
  out6 : Outport  Port=7
  out7 : Outport  Port=8
  out8 : Outport  Port=9
  wires:
  in8/1 -> delay8/1, adder_tree8/2(din_1)
  sync_in/1 -> adder_tree1/1(sync)
  in1/1 -> adder_tree1/2(din_1), adder_tree2/3(din_2)
  delay8/1 -> adder_tree1/3(din_2)  "d8"
  adder_tree1/2(dout) -> out1/1
  adder_tree1/1(sync_out) -> adder_tree2/1(sync)  "adder_tree_sync_in1"
  in2/1 -> adder_tree2/2(din_1), adder_tree3/3(din_2)
  adder_tree2/2(dout) -> out2/1
  adder_tree2/1(sync_out) -> adder_tree3/1(sync)  "adder_tree_sync_in2"
  in3/1 -> adder_tree3/2(din_1), adder_tree4/3(din_2)
  adder_tree3/2(dout) -> out3/1
  adder_tree3/1(sync_out) -> adder_tree4/1(sync)  "adder_tree_sync_in3"
  in4/1 -> adder_tree4/2(din_1), adder_tree5/3(din_2)
  adder_tree4/2(dout) -> out4/1
  adder_tree4/1(sync_out) -> adder_tree5/1(sync)  "adder_tree_sync_in4"
  in5/1 -> adder_tree5/2(din_1), adder_tree6/3(din_2)
  adder_tree5/2(dout) -> out5/1
  adder_tree5/1(sync_out) -> adder_tree6/1(sync)  "adder_tree_sync_in5"
  in6/1 -> adder_tree6/2(din_1), adder_tree7/3(din_2)
  adder_tree6/2(dout) -> out6/1
  adder_tree6/1(sync_out) -> adder_tree7/1(sync)  "adder_tree_sync_in6"
  in7/1 -> adder_tree7/2(din_1), adder_tree8/3(din_2)
  adder_tree7/2(dout) -> out7/1
  adder_tree7/1(sync_out) -> adder_tree8/1(sync)  "adder_tree_sync_in7"
  adder_tree8/2(dout) -> out8/1
  adder_tree8/1(sync_out) -> sync_out/1  "adder_tree_sync_in8"

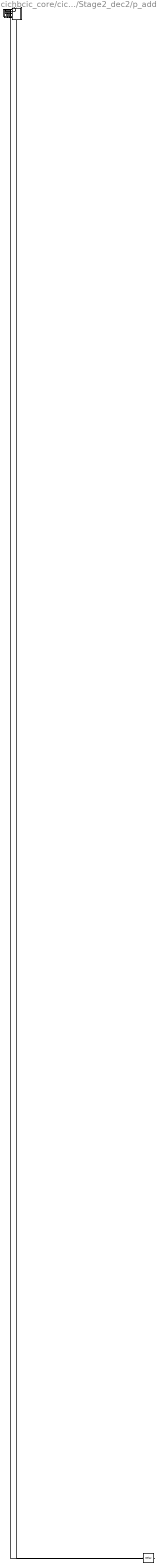
== system cichbcic_core/cic_pow2_1/Stage2_dec2/p_adder3 ==
  sync_in : Inport
  in1 : Inport  Port=2
  in2 : Inport  Port=3
  in3 : Inport  Port=4
  in4 : Inport  Port=5
  in5 : Inport  Port=6
  in6 : Inport  Port=7
  in7 : Inport  Port=8
  in8 : Inport  Port=9
  adder_tree1 : Subsystem
  adder_tree2 : Subsystem
  adder_tree3 : Subsystem
  adder_tree4 : Subsystem
  adder_tree5 : Subsystem
  adder_tree6 : Subsystem
  adder_tree7 : Subsystem
  adder_tree8 : Subsystem
  delay8 : xbsIndex_r4/Delay  rst=off  infoeditControl=Selection of Reset will increase slice count due to use of real FFs and instead of SRLs  en=off  latency=1  dbl_ovrd=off  reg_retiming=off  block_type=delay
  sync_out : Outport
  out1 : Outport  Port=2
  out2 : Outport  Port=3
  out3 : Outport  Port=4
  out4 : Outport  Port=5
  out5 : Outport  Port=6
  out6 : Outport  Port=7
  out7 : Outport  Port=8
  out8 : Outport  Port=9
  wires:
  in8/1 -> delay8/1, adder_tree8/2(din_1)
  sync_in/1 -> adder_tree1/1(sync)
  in1/1 -> adder_tree1/2(din_1), adder_tree2/3(din_2)
  delay8/1 -> adder_tree1/3(din_2)  "d8"
  adder_tree1/2(dout) -> out1/1
  adder_tree1/1(sync_out) -> adder_tree2/1(sync)  "adder_tree_sync_in1"
  in2/1 -> adder_tree2/2(din_1), adder_tree3/3(din_2)
  adder_tree2/2(dout) -> out2/1
  adder_tree2/1(sync_out) -> adder_tree3/1(sync)  "adder_tree_sync_in2"
  in3/1 -> adder_tree3/2(din_1), adder_tree4/3(din_2)
  adder_tree3/2(dout) -> out3/1
  adder_tree3/1(sync_out) -> adder_tree4/1(sync)  "adder_tree_sync_in3"
  in4/1 -> adder_tree4/2(din_1), adder_tree5/3(din_2)
  adder_tree4/2(dout) -> out4/1
  adder_tree4/1(sync_out) -> adder_tree5/1(sync)  "adder_tree_sync_in4"
  in5/1 -> adder_tree5/2(din_1), adder_tree6/3(din_2)
  adder_tree5/2(dout) -> out5/1
  adder_tree5/1(sync_out) -> adder_tree6/1(sync)  "adder_tree_sync_in5"
  in6/1 -> adder_tree6/2(din_1), adder_tree7/3(din_2)
  adder_tree6/2(dout) -> out6/1
  adder_tree6/1(sync_out) -> adder_tree7/1(sync)  "adder_tree_sync_in6"
  in7/1 -> adder_tree7/2(din_1), adder_tree8/3(din_2)
  adder_tree7/2(dout) -> out7/1
  adder_tree7/1(sync_out) -> adder_tree8/1(sync)  "adder_tree_sync_in7"
  adder_tree8/2(dout) -> out8/1
  adder_tree8/1(sync_out) -> sync_out/1  "adder_tree_sync_in8"

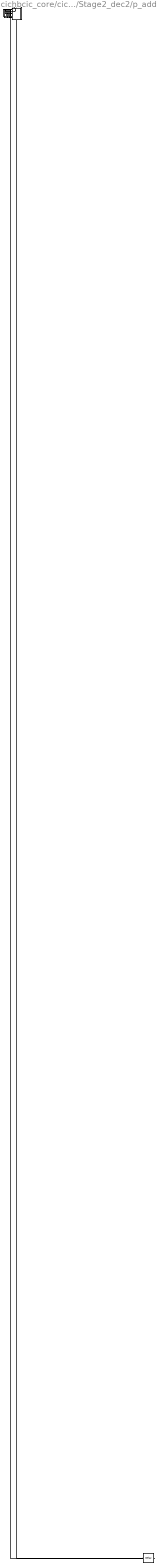
== system cichbcic_core/cic_pow2_1/Stage2_dec2/p_adder4 ==
  sync_in : Inport
  in1 : Inport  Port=2
  in2 : Inport  Port=3
  in3 : Inport  Port=4
  in4 : Inport  Port=5
  in5 : Inport  Port=6
  in6 : Inport  Port=7
  in7 : Inport  Port=8
  in8 : Inport  Port=9
  adder_tree1 : Subsystem
  adder_tree2 : Subsystem
  adder_tree3 : Subsystem
  adder_tree4 : Subsystem
  adder_tree5 : Subsystem
  adder_tree6 : Subsystem
  adder_tree7 : Subsystem
  adder_tree8 : Subsystem
  delay8 : xbsIndex_r4/Delay  rst=off  infoeditControl=Selection of Reset will increase slice count due to use of real FFs and instead of SRLs  en=off  latency=1  dbl_ovrd=off  reg_retiming=off  block_type=delay
  sync_out : Outport
  out1 : Outport  Port=2
  out2 : Outport  Port=3
  out3 : Outport  Port=4
  out4 : Outport  Port=5
  out5 : Outport  Port=6
  out6 : Outport  Port=7
  out7 : Outport  Port=8
  out8 : Outport  Port=9
  wires:
  in8/1 -> delay8/1, adder_tree8/2(din_1)
  sync_in/1 -> adder_tree1/1(sync)
  in1/1 -> adder_tree1/2(din_1), adder_tree2/3(din_2)
  delay8/1 -> adder_tree1/3(din_2)  "d8"
  adder_tree1/2(dout) -> out1/1
  adder_tree1/1(sync_out) -> adder_tree2/1(sync)  "adder_tree_sync_in1"
  in2/1 -> adder_tree2/2(din_1), adder_tree3/3(din_2)
  adder_tree2/2(dout) -> out2/1
  adder_tree2/1(sync_out) -> adder_tree3/1(sync)  "adder_tree_sync_in2"
  in3/1 -> adder_tree3/2(din_1), adder_tree4/3(din_2)
  adder_tree3/2(dout) -> out3/1
  adder_tree3/1(sync_out) -> adder_tree4/1(sync)  "adder_tree_sync_in3"
  in4/1 -> adder_tree4/2(din_1), adder_tree5/3(din_2)
  adder_tree4/2(dout) -> out4/1
  adder_tree4/1(sync_out) -> adder_tree5/1(sync)  "adder_tree_sync_in4"
  in5/1 -> adder_tree5/2(din_1), adder_tree6/3(din_2)
  adder_tree5/2(dout) -> out5/1
  adder_tree5/1(sync_out) -> adder_tree6/1(sync)  "adder_tree_sync_in5"
  in6/1 -> adder_tree6/2(din_1), adder_tree7/3(din_2)
  adder_tree6/2(dout) -> out6/1
  adder_tree6/1(sync_out) -> adder_tree7/1(sync)  "adder_tree_sync_in6"
  in7/1 -> adder_tree7/2(din_1), adder_tree8/3(din_2)
  adder_tree7/2(dout) -> out7/1
  adder_tree7/1(sync_out) -> adder_tree8/1(sync)  "adder_tree_sync_in7"
  adder_tree8/2(dout) -> out8/1
  adder_tree8/1(sync_out) -> sync_out/1  "adder_tree_sync_in8"

== system cichbcic_core/cic_pow2_1/Stage3_dec2/p_adder1 ==
  sync_in : Inport
  in1 : Inport  Port=2
  in2 : Inport  Port=3
  in3 : Inport  Port=4
  in4 : Inport  Port=5
  adder_tree1 : Subsystem
  adder_tree2 : Subsystem
  adder_tree3 : Subsystem
  adder_tree4 : Subsystem
  delay4 : xbsIndex_r4/Delay  rst=off  infoeditControl=Selection of Reset will increase slice count due to use of real FFs and instead of SRLs  en=off  latency=1  dbl_ovrd=off  reg_retiming=off  block_type=delay
  sync_out : Outport
  out1 : Outport  Port=2
  out2 : Outport  Port=3
  out3 : Outport  Port=4
  out4 : Outport  Port=5
  wires:
  in4/1 -> delay4/1, adder_tree4/2(din_1)
  sync_in/1 -> adder_tree1/1(sync)
  in1/1 -> adder_tree1/2(din_1), adder_tree2/3(din_2)
  delay4/1 -> adder_tree1/3(din_2)  "d4"
  adder_tree1/2(dout) -> out1/1
  adder_tree1/1(sync_out) -> adder_tree2/1(sync)  "adder_tree_sync_in1"
  in2/1 -> adder_tree2/2(din_1), adder_tree3/3(din_2)
  adder_tree2/2(dout) -> out2/1
  adder_tree2/1(sync_out) -> adder_tree3/1(sync)  "adder_tree_sync_in2"
  in3/1 -> adder_tree3/2(din_1), adder_tree4/3(din_2)
  adder_tree3/2(dout) -> out3/1
  adder_tree3/1(sync_out) -> adder_tree4/1(sync)  "adder_tree_sync_in3"
  adder_tree4/2(dout) -> out4/1
  adder_tree4/1(sync_out) -> sync_out/1  "adder_tree_sync_in4"

== system cichbcic_core/cic_pow2_1/Stage3_dec2/p_adder2 ==
  sync_in : Inport
  in1 : Inport  Port=2
  in2 : Inport  Port=3
  in3 : Inport  Port=4
  in4 : Inport  Port=5
  adder_tree1 : Subsystem
  adder_tree2 : Subsystem
  adder_tree3 : Subsystem
  adder_tree4 : Subsystem
  delay4 : xbsIndex_r4/Delay  rst=off  infoeditControl=Selection of Reset will increase slice count due to use of real FFs and instead of SRLs  en=off  latency=1  dbl_ovrd=off  reg_retiming=off  block_type=delay
  sync_out : Outport
  out1 : Outport  Port=2
  out2 : Outport  Port=3
  out3 : Outport  Port=4
  out4 : Outport  Port=5
  wires:
  in4/1 -> delay4/1, adder_tree4/2(din_1)
  sync_in/1 -> adder_tree1/1(sync)
  in1/1 -> adder_tree1/2(din_1), adder_tree2/3(din_2)
  delay4/1 -> adder_tree1/3(din_2)  "d4"
  adder_tree1/2(dout) -> out1/1
  adder_tree1/1(sync_out) -> adder_tree2/1(sync)  "adder_tree_sync_in1"
  in2/1 -> adder_tree2/2(din_1), adder_tree3/3(din_2)
  adder_tree2/2(dout) -> out2/1
  adder_tree2/1(sync_out) -> adder_tree3/1(sync)  "adder_tree_sync_in2"
  in3/1 -> adder_tree3/2(din_1), adder_tree4/3(din_2)
  adder_tree3/2(dout) -> out3/1
  adder_tree3/1(sync_out) -> adder_tree4/1(sync)  "adder_tree_sync_in3"
  adder_tree4/2(dout) -> out4/1
  adder_tree4/1(sync_out) -> sync_out/1  "adder_tree_sync_in4"

== system cichbcic_core/cic_pow2_1/Stage3_dec2/p_adder3 ==
  sync_in : Inport
  in1 : Inport  Port=2
  in2 : Inport  Port=3
  in3 : Inport  Port=4
  in4 : Inport  Port=5
  adder_tree1 : Subsystem
  adder_tree2 : Subsystem
  adder_tree3 : Subsystem
  adder_tree4 : Subsystem
  delay4 : xbsIndex_r4/Delay  rst=off  infoeditControl=Selection of Reset will increase slice count due to use of real FFs and instead of SRLs  en=off  latency=1  dbl_ovrd=off  reg_retiming=off  block_type=delay
  sync_out : Outport
  out1 : Outport  Port=2
  out2 : Outport  Port=3
  out3 : Outport  Port=4
  out4 : Outport  Port=5
  wires:
  in4/1 -> delay4/1, adder_tree4/2(din_1)
  sync_in/1 -> adder_tree1/1(sync)
  in1/1 -> adder_tree1/2(din_1), adder_tree2/3(din_2)
  delay4/1 -> adder_tree1/3(din_2)  "d4"
  adder_tree1/2(dout) -> out1/1
  adder_tree1/1(sync_out) -> adder_tree2/1(sync)  "adder_tree_sync_in1"
  in2/1 -> adder_tree2/2(din_1), adder_tree3/3(din_2)
  adder_tree2/2(dout) -> out2/1
  adder_tree2/1(sync_out) -> adder_tree3/1(sync)  "adder_tree_sync_in2"
  in3/1 -> adder_tree3/2(din_1), adder_tree4/3(din_2)
  adder_tree3/2(dout) -> out3/1
  adder_tree3/1(sync_out) -> adder_tree4/1(sync)  "adder_tree_sync_in3"
  adder_tree4/2(dout) -> out4/1
  adder_tree4/1(sync_out) -> sync_out/1  "adder_tree_sync_in4"

== system cichbcic_core/cic_pow2_1/Stage3_dec2/p_adder4 ==
  sync_in : Inport
  in1 : Inport  Port=2
  in2 : Inport  Port=3
  in3 : Inport  Port=4
  in4 : Inport  Port=5
  adder_tree1 : Subsystem
  adder_tree2 : Subsystem
  adder_tree3 : Subsystem
  adder_tree4 : Subsystem
  delay4 : xbsIndex_r4/Delay  rst=off  infoeditControl=Selection of Reset will increase slice count due to use of real FFs and instead of SRLs  en=off  latency=1  dbl_ovrd=off  reg_retiming=off  block_type=delay
  sync_out : Outport
  out1 : Outport  Port=2
  out2 : Outport  Port=3
  out3 : Outport  Port=4
  out4 : Outport  Port=5
  wires:
  in4/1 -> delay4/1, adder_tree4/2(din_1)
  sync_in/1 -> adder_tree1/1(sync)
  in1/1 -> adder_tree1/2(din_1), adder_tree2/3(din_2)
  delay4/1 -> adder_tree1/3(din_2)  "d4"
  adder_tree1/2(dout) -> out1/1
  adder_tree1/1(sync_out) -> adder_tree2/1(sync)  "adder_tree_sync_in1"
  in2/1 -> adder_tree2/2(din_1), adder_tree3/3(din_2)
  adder_tree2/2(dout) -> out2/1
  adder_tree2/1(sync_out) -> adder_tree3/1(sync)  "adder_tree_sync_in2"
  in3/1 -> adder_tree3/2(din_1), adder_tree4/3(din_2)
  adder_tree3/2(dout) -> out3/1
  adder_tree3/1(sync_out) -> adder_tree4/1(sync)  "adder_tree_sync_in3"
  adder_tree4/2(dout) -> out4/1
  adder_tree4/1(sync_out) -> sync_out/1  "adder_tree_sync_in4"

== system cichbcic_core/cic_pow2_1/Stage4_dec2/p_adder1 ==
  sync_in : Inport
  in1 : Inport  Port=2
  in2 : Inport  Port=3
  adder_tree1 : Subsystem
  adder_tree2 : Subsystem
  delay2 : xbsIndex_r4/Delay  rst=off  infoeditControl=Selection of Reset will increase slice count due to use of real FFs and instead of SRLs  en=off  latency=1  dbl_ovrd=off  reg_retiming=off  block_type=delay
  sync_out : Outport
  out1 : Outport  Port=2
  out2 : Outport  Port=3
  wires:
  in2/1 -> delay2/1, adder_tree2/2(din_1)
  sync_in/1 -> adder_tree1/1(sync)
  in1/1 -> adder_tree1/2(din_1), adder_tree2/3(din_2)
  delay2/1 -> adder_tree1/3(din_2)  "d2"
  adder_tree1/2(dout) -> out1/1
  adder_tree1/1(sync_out) -> adder_tree2/1(sync)  "adder_tree_sync_in1"
  adder_tree2/2(dout) -> out2/1
  adder_tree2/1(sync_out) -> sync_out/1  "adder_tree_sync_in2"

== system cichbcic_core/cic_pow2_1/Stage4_dec2/p_adder2 ==
  sync_in : Inport
  in1 : Inport  Port=2
  in2 : Inport  Port=3
  adder_tree1 : Subsystem
  adder_tree2 : Subsystem
  delay2 : xbsIndex_r4/Delay  rst=off  infoeditControl=Selection of Reset will increase slice count due to use of real FFs and instead of SRLs  en=off  latency=1  dbl_ovrd=off  reg_retiming=off  block_type=delay
  sync_out : Outport
  out1 : Outport  Port=2
  out2 : Outport  Port=3
  wires:
  in2/1 -> delay2/1, adder_tree2/2(din_1)
  sync_in/1 -> adder_tree1/1(sync)
  in1/1 -> adder_tree1/2(din_1), adder_tree2/3(din_2)
  delay2/1 -> adder_tree1/3(din_2)  "d2"
  adder_tree1/2(dout) -> out1/1
  adder_tree1/1(sync_out) -> adder_tree2/1(sync)  "adder_tree_sync_in1"
  adder_tree2/2(dout) -> out2/1
  adder_tree2/1(sync_out) -> sync_out/1  "adder_tree_sync_in2"

== system cichbcic_core/cic_pow2_1/Stage4_dec2/p_adder3 ==
  sync_in : Inport
  in1 : Inport  Port=2
  in2 : Inport  Port=3
  adder_tree1 : Subsystem
  adder_tree2 : Subsystem
  delay2 : xbsIndex_r4/Delay  rst=off  infoeditControl=Selection of Reset will increase slice count due to use of real FFs and instead of SRLs  en=off  latency=1  dbl_ovrd=off  reg_retiming=off  block_type=delay
  sync_out : Outport
  out1 : Outport  Port=2
  out2 : Outport  Port=3
  wires:
  in2/1 -> delay2/1, adder_tree2/2(din_1)
  sync_in/1 -> adder_tree1/1(sync)
  in1/1 -> adder_tree1/2(din_1), adder_tree2/3(din_2)
  delay2/1 -> adder_tree1/3(din_2)  "d2"
  adder_tree1/2(dout) -> out1/1
  adder_tree1/1(sync_out) -> adder_tree2/1(sync)  "adder_tree_sync_in1"
  adder_tree2/2(dout) -> out2/1
  adder_tree2/1(sync_out) -> sync_out/1  "adder_tree_sync_in2"

== system cichbcic_core/cic_pow2_1/Stage4_dec2/p_adder4 ==
  sync_in : Inport
  in1 : Inport  Port=2
  in2 : Inport  Port=3
  adder_tree1 : Subsystem
  adder_tree2 : Subsystem
  delay2 : xbsIndex_r4/Delay  rst=off  infoeditControl=Selection of Reset will increase slice count due to use of real FFs and instead of SRLs  en=off  latency=1  dbl_ovrd=off  reg_retiming=off  block_type=delay
  sync_out : Outport
  out1 : Outport  Port=2
  out2 : Outport  Port=3
  wires:
  in2/1 -> delay2/1, adder_tree2/2(din_1)
  sync_in/1 -> adder_tree1/1(sync)
  in1/1 -> adder_tree1/2(din_1), adder_tree2/3(din_2)
  delay2/1 -> adder_tree1/3(din_2)  "d2"
  adder_tree1/2(dout) -> out1/1
  adder_tree1/1(sync_out) -> adder_tree2/1(sync)  "adder_tree_sync_in1"
  adder_tree2/2(dout) -> out2/1
  adder_tree2/1(sync_out) -> sync_out/1  "adder_tree_sync_in2"

== system cichbcic_core/cic_pow2_1/Stage5_dec2/Down_sample1 ==
  In : Inport
  sync_in : Inport  Port=2
  Register : xbsIndex_r4/Register  init=0  rst=off  en=on  dbl_ovrd=off  block_type=register
  en_gen : Subsystem
      settings: AttributesFormatString=|
      | hold period: 2
      | explicit clk period:on , input clk period:1
  sync_delay : xbsIndex_r4/Delay  rst=off  infoeditControl=Selection of Reset will increase slice count due to use of real FFs and instead of SRLs  en=off  latency=1  dbl_ovrd=off  reg_retiming=off  block_type=delay
  Out : Outport
  sync_out : Outport  Port=2
  wires:
  sync_in/1 -> en_gen/1(sync_in), sync_delay/1
  In/1 -> Register/1
  en_gen/1(en_out) -> Register/2  "en"
  Register/1 -> Out/1
  sync_delay/1 -> sync_out/1

== system cichbcic_core/cic_pow2_1/Stage5_dec2/adder_tree1 ==
  sync : Inport
  din_1 : Inport  Port=2
  din_2 : Inport  Port=3
  adder_0 : xbsIndex_r4/AddSub  mode=Addition  use_carryin=off  use_carryout=off  en=off  latency=1  precision=Full  arith_type=Unsigned  n_bits=18  bin_pt=17  quantization="Round  (unbiased: +/- Inf)"  overflow=Saturate  dbl_ovrd=off  use_behavioral_HDL=on  hw_selection=Fabric  pipelined=off  block_type=addsub
  sync_delay : xbsIndex_r4/Delay  rst=off  infoeditControl=Selection of Reset will increase slice count due to use of real FFs and instead of SRLs  en=off  latency=1  dbl_ovrd=off  reg_retiming=off  block_type=delay
  sync_out : Outport
  dout : Outport  Port=2
  wires:
  sync/1 -> sync_delay/1
  sync_delay/1 -> sync_out/1
  din_2/1 -> adder_0/1
  din_1/1 -> adder_0/2
  adder_0/1 -> dout/1

== system cichbcic_core/cic_pow2_1/Stage5_dec2/adder_tree2 ==
  sync : Inport
  din_1 : Inport  Port=2
  din_2 : Inport  Port=3
  adder_0 : xbsIndex_r4/AddSub  mode=Addition  use_carryin=off  use_carryout=off  en=off  latency=1  precision=Full  arith_type=Unsigned  n_bits=18  bin_pt=17  quantization="Round  (unbiased: +/- Inf)"  overflow=Saturate  dbl_ovrd=off  use_behavioral_HDL=on  hw_selection=Fabric  pipelined=off  block_type=addsub
  sync_delay : xbsIndex_r4/Delay  rst=off  infoeditControl=Selection of Reset will increase slice count due to use of real FFs and instead of SRLs  en=off  latency=1  dbl_ovrd=off  reg_retiming=off  block_type=delay
  sync_out : Outport
  dout : Outport  Port=2
  wires:
  sync/1 -> sync_delay/1
  sync_delay/1 -> sync_out/1
  din_2/1 -> adder_0/1
  din_1/1 -> adder_0/2
  adder_0/1 -> dout/1

== system cichbcic_core/cic_pow2_1/Stage5_dec2/adder_tree3 ==
  sync : Inport
  din_1 : Inport  Port=2
  din_2 : Inport  Port=3
  adder_0 : xbsIndex_r4/AddSub  mode=Addition  use_carryin=off  use_carryout=off  en=off  latency=1  precision=Full  arith_type=Unsigned  n_bits=18  bin_pt=17  quantization="Round  (unbiased: +/- Inf)"  overflow=Saturate  dbl_ovrd=off  use_behavioral_HDL=on  hw_selection=Fabric  pipelined=off  block_type=addsub
  sync_delay : xbsIndex_r4/Delay  rst=off  infoeditControl=Selection of Reset will increase slice count due to use of real FFs and instead of SRLs  en=off  latency=1  dbl_ovrd=off  reg_retiming=off  block_type=delay
  sync_out : Outport
  dout : Outport  Port=2
  wires:
  sync/1 -> sync_delay/1
  sync_delay/1 -> sync_out/1
  din_2/1 -> adder_0/1
  din_1/1 -> adder_0/2
  adder_0/1 -> dout/1

== system cichbcic_core/cic_pow2_1/Stage5_dec2/adder_tree4 ==
  sync : Inport
  din_1 : Inport  Port=2
  din_2 : Inport  Port=3
  adder_0 : xbsIndex_r4/AddSub  mode=Addition  use_carryin=off  use_carryout=off  en=off  latency=1  precision=Full  arith_type=Unsigned  n_bits=18  bin_pt=17  quantization="Round  (unbiased: +/- Inf)"  overflow=Saturate  dbl_ovrd=off  use_behavioral_HDL=on  hw_selection=Fabric  pipelined=off  block_type=addsub
  sync_delay : xbsIndex_r4/Delay  rst=off  infoeditControl=Selection of Reset will increase slice count due to use of real FFs and instead of SRLs  en=off  latency=1  dbl_ovrd=off  reg_retiming=off  block_type=delay
  sync_out : Outport
  dout : Outport  Port=2
  wires:
  sync/1 -> sync_delay/1
  sync_delay/1 -> sync_out/1
  din_2/1 -> adder_0/1
  din_1/1 -> adder_0/2
  adder_0/1 -> dout/1

== system cichbcic_core/cic_stage_dec3/Down_sample1/en_gen ==
  sync_in : Inport
  Constant : xbsIndex_r4/Constant  const=0  gui_display_data_type=Fixed-point  arith_type=Signed (2's comp)  n_bits=16  bin_pt=14  preci_type=Single  exp_width=8  frac_width=24  explicit_period=off  period=1  equ=P=C  opselect=C  inp2=PCIN>>17  opr=+  inp1=P  carry=CIN  dbl_ovrd=off  block_type=constant
  Counter1 : xbsIndex_r4/Counter  cnt_type=Count Limited  cnt_to=0  operation=Down  start_count=7  cnt_by_val=1  arith_type=Unsigned  n_bits=3  bin_pt=0  load_pin=off  rst=on  en=off  explicit_period=on  period=1  dbl_ovrd=off  use_behavioral_HDL=off  implementation=Fabric  block_type=counter
  Logical : xbsIndex_r4/Logical  logical_function=OR  inputs=2  en=off  latency=0  precision=Full  arith_type=Unsigned  n_bits=16  bin_pt=0  align_bp=on  dbl_ovrd=off  block_type=logical
  Relational : xbsIndex_r4/Relational  mode=a=b  en=off  latency=0  dbl_ovrd=off  block_type=relational
  en_out : Outport
  wires:
  sync_in/1 -> Logical/2
  Logical/1 -> Counter1/1, en_out/1  "xlsub1_Logical_out1"
  Counter1/1 -> Relational/1  "xlsub1_Counter1_out1"
  Constant/1 -> Relational/2  "xlsub1_Constant_out1"
  Relational/1 -> Logical/1  "xlsub1_Relational_out1"

== system cichbcic_core/cic_stage_dec4/Down_sample1/en_gen ==
  sync_in : Inport
  Constant : xbsIndex_r4/Constant  const=0  gui_display_data_type=Fixed-point  arith_type=Signed (2's comp)  n_bits=16  bin_pt=14  preci_type=Single  exp_width=8  frac_width=24  explicit_period=off  period=1  equ=P=C  opselect=C  inp2=PCIN>>17  opr=+  inp1=P  carry=CIN  dbl_ovrd=off  block_type=constant
  Counter1 : xbsIndex_r4/Counter  cnt_type=Count Limited  cnt_to=0  operation=Down  start_count=3  cnt_by_val=1  arith_type=Unsigned  n_bits=2  bin_pt=0  load_pin=off  rst=on  en=off  explicit_period=on  period=1  dbl_ovrd=off  use_behavioral_HDL=off  implementation=Fabric  block_type=counter
  Logical : xbsIndex_r4/Logical  logical_function=OR  inputs=2  en=off  latency=0  precision=Full  arith_type=Unsigned  n_bits=16  bin_pt=0  align_bp=on  dbl_ovrd=off  block_type=logical
  Relational : xbsIndex_r4/Relational  mode=a=b  en=off  latency=0  dbl_ovrd=off  block_type=relational
  en_out : Outport
  wires:
  sync_in/1 -> Logical/2
  Logical/1 -> Counter1/1, en_out/1  "xlsub1_Logical_out1"
  Counter1/1 -> Relational/1  "xlsub1_Counter1_out1"
  Constant/1 -> Relational/2  "xlsub1_Constant_out1"
  Relational/1 -> Logical/1  "xlsub1_Relational_out1"

== system cichbcic_core/cic_pow2_1/Stage1_dec2/p_adder1/adder_tree1 ==
  sync : Inport
  din_1 : Inport  Port=2
  din_2 : Inport  Port=3
  adder_0 : xbsIndex_r4/AddSub  mode=Addition  use_carryin=off  use_carryout=off  en=off  latency=1  precision=Full  arith_type=Unsigned  n_bits=18  bin_pt=17  quantization="Round  (unbiased: +/- Inf)"  overflow=Saturate  dbl_ovrd=off  use_behavioral_HDL=on  hw_selection=Fabric  pipelined=off  block_type=addsub
  sync_delay : xbsIndex_r4/Delay  rst=off  infoeditControl=Selection of Reset will increase slice count due to use of real FFs and instead of SRLs  en=off  latency=1  dbl_ovrd=off  reg_retiming=off  block_type=delay
  sync_out : Outport
  dout : Outport  Port=2
  wires:
  sync/1 -> sync_delay/1
  sync_delay/1 -> sync_out/1
  din_2/1 -> adder_0/1
  din_1/1 -> adder_0/2
  adder_0/1 -> dout/1

== system cichbcic_core/cic_pow2_1/Stage1_dec2/p_adder1/adder_tree10 ==
  sync : Inport
  din_1 : Inport  Port=2
  din_2 : Inport  Port=3
  adder_0 : xbsIndex_r4/AddSub  mode=Addition  use_carryin=off  use_carryout=off  en=off  latency=1  precision=Full  arith_type=Unsigned  n_bits=18  bin_pt=17  quantization="Round  (unbiased: +/- Inf)"  overflow=Saturate  dbl_ovrd=off  use_behavioral_HDL=on  hw_selection=Fabric  pipelined=off  block_type=addsub
  sync_delay : xbsIndex_r4/Delay  rst=off  infoeditControl=Selection of Reset will increase slice count due to use of real FFs and instead of SRLs  en=off  latency=1  dbl_ovrd=off  reg_retiming=off  block_type=delay
  sync_out : Outport
  dout : Outport  Port=2
  wires:
  sync/1 -> sync_delay/1
  sync_delay/1 -> sync_out/1
  din_2/1 -> adder_0/1
  din_1/1 -> adder_0/2
  adder_0/1 -> dout/1
